simulink model "across_object"  (R2016b)
settings: Solver=FixedStepAuto  StartTime=0.0  StopTime=10.0  FixedStep=0.025  RelTol=1e-3
settings Model: Creator=Administrator  LastModifiedBy=Administrator

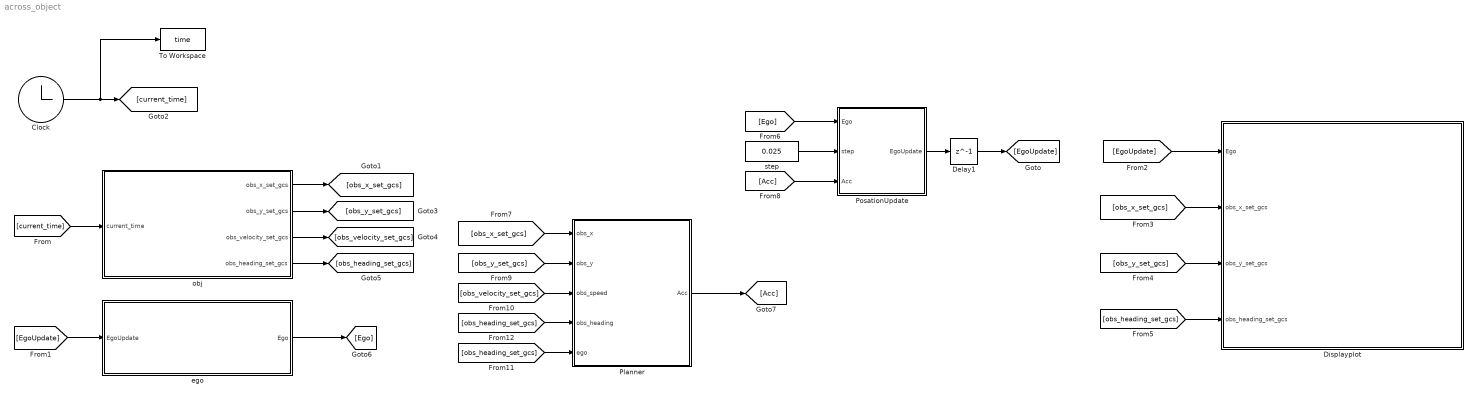
== system across_object ==
  Clock : Clock
  Delay1 : Delay  DelayLength=1  InitialCondition=0
  Displayplot : MATLAB Function  TreatAsAtomicUnit=on
  Planner : Subsystem
  PosationUpdate : MATLAB Function  TreatAsAtomicUnit=on
  To Workspace : ToWorkspace  VariableName=time  SampleTime=-1
  ego : MATLAB Function  TreatAsAtomicUnit=on
  obj : MATLAB Function  TreatAsAtomicUnit=on
  "step " : Constant  Value=0.025
  wires:
  Clock/1 -> To Workspace/1, [current_time]
  [current_time] -> obj/1(current_time)
  PosationUpdate/1(EgoUpdate) -> Delay1/1
  Delay1/1 -> [EgoUpdate]
  [EgoUpdate] -> ego/1(EgoUpdate)
  [EgoUpdate] -> Displayplot/1(Ego)
  obj/1(obs_x_set_gcs) -> [obs_x_set_gcs]
  obj/2(obs_y_set_gcs) -> [obs_y_set_gcs]
  obj/3(obs_velocity_set_gcs) -> [obs_velocity_set_gcs]
  obj/4(obs_heading_set_gcs) -> [obs_heading_set_gcs]
  [obs_x_set_gcs] -> Displayplot/2(obs_x_set_gcs)
  [obs_y_set_gcs] -> Displayplot/3(obs_y_set_gcs)
  [obs_heading_set_gcs] -> Displayplot/4(obs_heading_set_gcs)
  "step "/1 -> PosationUpdate/2(step)
  ego/1(Ego) -> [Ego]
  [Ego] -> PosationUpdate/1(Ego)
  [obs_x_set_gcs] -> Planner/1(obs_x)
  Planner/1(Acc) -> [Acc]
  [Acc] -> PosationUpdate/3(Acc)
  [obs_y_set_gcs] -> Planner/2(obs_y)
  [obs_velocity_set_gcs] -> Planner/3(obs_speed)
  [obs_heading_set_gcs] -> Planner/5(ego)
  [obs_heading_set_gcs] -> Planner/4(obs_heading)

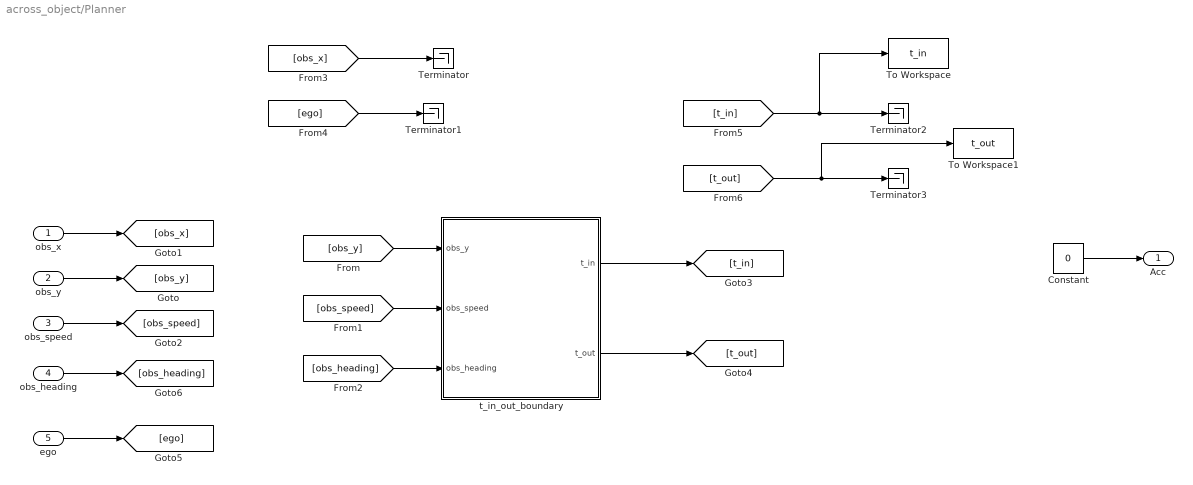
== system across_object/Planner ==
  obs_x : Inport
  obs_y : Inport  Port=2
  obs_speed : Inport  Port=3
  obs_heading : Inport  Port=4
  ego : Inport  Port=5
  Constant : Constant  Value=0
  Terminator{,1..3} (4 alike) : Terminator
  To Workspace : ToWorkspace  VariableName=t_in  SampleTime=-1
  To Workspace1 : ToWorkspace  VariableName=t_out  SampleTime=-1
  t_in_out_boundary : MATLAB Function  TreatAsAtomicUnit=on
  Acc : Outport
  wires:
  Constant/1 -> Acc/1
  obs_x/1 -> [obs_x]
  obs_y/1 -> [obs_y]
  obs_speed/1 -> [obs_speed]
  ego/1 -> [ego]
  [obs_y] -> t_in_out_boundary/1(obs_y)
  [obs_speed] -> t_in_out_boundary/2(obs_speed)
  t_in_out_boundary/1(t_in) -> [t_in]
  t_in_out_boundary/2(t_out) -> [t_out]
  obs_heading/1 -> [obs_heading]
  [obs_heading] -> t_in_out_boundary/3(obs_heading)
  [obs_x] -> Terminator/1
  [ego] -> Terminator1/1
  [t_in] -> To Workspace/1, Terminator2/1
  [t_out] -> To Workspace1/1, Terminator3/1

== matlab function across_object/ego ==
  data: EgoUpdate input Bus: Ego; Ego output Bus: Ego
function Ego = fcn(EgoUpdate)
persistent is_first_run
if isempty(is_first_run)
    is_first_run = 1;
end
if is_first_run > 0 %前10个周期没有规划轨迹 自车信息无法跟新
    is_first_run = is_first_run -1;
    Ego.x = 0;
    Ego.y = 0;     
    Ego.a = 0;
    Ego.speed = 5;
else
    Ego.x = EgoUpdate.x;
    Ego.y = EgoUpdate.y;     
    Ego.a = EgoUpdate.a;
    Ego.speed = EgoUpdate.speed;
end

== matlab function across_object/PosationUpdate ==
  data: Ego input Bus: Ego; step input; EgoUpdate output Bus: Ego; Acc input
function EgoUpdate = fcn(Ego,step,Acc)
    EgoUpdate.x = Ego.x + Ego.speed * step + 0.5*Acc*step^2;
    EgoUpdate.y = 0;     
    EgoUpdate.a = Acc;
    EgoUpdate.speed =  Ego.speed + Acc*step;
end

== matlab function across_object/Planner/t_in_out_boundary ==
  data: obs_y input; t_in output; obs_speed input; t_out output; obs_heading input
function [t_in,t_out] = fcn(obs_y,obs_speed,obs_heading)
LaneWidth = 4 ;%车道宽度4米  有车道线按照车道线计算  没有按照道路宽度6米计算 
ObjWidth = 2;%目标车长5米 宽2米
ObjLength = 5;
obj_lat_velocity = max(obs_speed,0.5);%目标车速 5kp - 45kph
obj_lat_head_pos = obs_y - ObjLength/2;%车头位置  obs_y左正右负

obj_global_heading = 0;%以自车坐标系不为中心  从左向右 0度 范围-45~45  从右向左 135 ~ 180  -180~ -135

if obj_global_heading >= -45/180*pi && obj_global_heading <= 45/180*pi
    AcrossType = uint8(1);%横穿类型从左到右
elseif obj_global_heading >= 135/180*pi && obj_global_heading <= -135/180*pi
    AcrossType = uint8(2);%横穿类型从右到左    
else
    AcrossType = uint8(0);%未知
end

if (obj_lat_head_pos >= 2 &&  AcrossType == uint8(1))|| (obj_lat_head_pos <= -2 &&  AcrossType == uint8(2))% 目标车在车道外
    t_in = (obj_lat_head_pos/obj_lat_velocity);
    if AcrossType == uint8(1)
        obj_lat_across_distance = obj_lat_head_pos + LaneWidth + ObjLength + 2;%目标车out的距离 加一个distanceoffset
        t_out = (obj_lat_across_distance/obj_lat_velocity);
    else
        obj_lat_across_distance = abs(obj_lat_head_pos) + LaneWidth + ObjLength + 2;%目标车out的距离 加一个distanceoffset
        t_out = (obj_lat_across_distance/obj_lat_velocity);
    end
elseif (obj_lat_head_pos >= (-LaneWidth/2 - ObjLength) &&  AcrossType == uint8(1)) || (obj_lat_head_pos >= (-LaneWidth/2 - ObjLength) &&  AcrossType == uint8(1)) % 目标车在车道里                                                                                          % 目标车在车道里
    t_in  = 0;
    if AcrossType == uint8(1)
        obj_lat_across_distance = obj_lat_head_pos + LaneWidth + ObjLength + 2;%目标车out的距离 加一个distanceoffset
        t_out = (obj_lat_across_distance/obj_lat_velocity);
    else
        obj_lat_across_distance =  LaneWidth + ObjLength + 2 - obj_lat_head_pos;%目标车out的距离 加一个distanceoffset
        t_out = (obj_lat_across_distance/obj_lat_velocity);
    end
else 
    t_in  = 500;%暂时给个无穷大
    t_out = 500;
end

== matlab function across_object/obj ==
  data: current_time input; obs_x_set_gcs output; obs_y_set_gcs output; obs_velocity_set_gcs output; obs_heading_set_gcs output
function [obs_x_set_gcs,obs_y_set_gcs,obs_velocity_set_gcs,obs_heading_set_gcs] = fcn(current_time)

% 动态障碍物 横穿道路
obs_x_set_gcs = 80;%
obs_y_set_gcs = 15 - 2*current_time;
obs_velocity_set_gcs = 2;
obs_heading_set_gcs= pi/2;

== matlab function across_object/Displayplot ==
  data: Ego input Bus: Ego; obs_x_set_gcs input; obs_y_set_gcs input; obs_heading_set_gcs input
function fcn(Ego,obs_x_set_gcs,obs_y_set_gcs,obs_heading_set_gcs)
coder.extrinsic('plot');
coder.extrinsic('patch');
coder.extrinsic('num2str');
%%定义道路宽度  
LaneWidth = 4;%
LaneLength = 800;%路长800米
global_path_x = 0: 0.2 : LaneLength;%
num1 = uint16(length(global_path_x));%计算多少个点
global_path_y = zeros(1,num1);
leftLaneMarker = global_path_y + LaneWidth;%左车道线的y坐标值
rightLaneMarker = global_path_y - LaneWidth; 
%%
%显示自车位置   %%绘制轨迹点
    plot(global_path_x,global_path_y,'b--',  global_path_x,leftLaneMarker,'k-', global_path_x,rightLaneMarker,'k-');
    
    EgoWidth = 2;%车宽
    EgoLength = 12;
    EgoPosX = Ego.x;
    EgoPosY = Ego.y;
    EgoHeading = 0;
    EgoColor = [0.9 0.9 0.9 0.9];
    Boxyx = zeros(1,4);
    Boxyy = zeros(1,4);
    Boxyx(1) = EgoPosX - EgoWidth/2*sin(EgoHeading);
    Boxyy(1) = EgoPosY + EgoWidth/2*cos(EgoHeading);
    Boxyx(2) = EgoPosX + EgoWidth/2*sin(EgoHeading);
    Boxyy(2) = EgoPosY - EgoWidth/2*cos(EgoHeading);
    Boxyx(3) = Boxyx(2) + EgoLength*cos(EgoHeading);
    Boxyy(3) = Boxyy(2) + EgoLength*sin(EgoHeading);
    Boxyx(4) = Boxyx(1) + EgoLength*cos(EgoHeading);
    Boxyy(4) = Boxyy(1) + EgoLength*sin(EgoHeading);
    patch(Boxyx,Boxyy,EgoColor);
    axis([EgoPosX-20,EgoPosX+120,-15,15]);%坐标范围
    text(EgoPosX,10,'EgoSpeed');
    text(EgoPosX+25,10,num2str(Ego.speed));
    text(EgoPosX,12,'EgoA');
    text(EgoPosX+25,12,num2str(Ego.a));
    
    objWidth = 7;
    objLength = 3;
    objPosX =obs_x_set_gcs;
    objPosY = obs_y_set_gcs;
    objHeading = obs_heading_set_gcs;
    objColor = [0.9 0.9 0.9 0.9];
    Boxyx(1) = objPosX - objWidth/2*sin(objHeading);
    Boxyy(1) = objPosY + objWidth/2*cos(objHeading);
    Boxyx(2) = objPosX + objWidth/2*sin(objHeading);
    Boxyy(2) = objPosY - objWidth/2*cos(objHeading);
    Boxyx(3) = Boxyx(2) + objLength*cos(objHeading);
    Boxyy(3) = Boxyy(2) + objLength*sin(objHeading);
    Boxyx(4) = Boxyx(1) + objLength*cos(objHeading);
    Boxyy(4) = Boxyy(1) + objLength*sin(objHeading);
    patch(Boxyx,Boxyy,objColor);
